simulink model "sus"  (Simulink 6.5)
settings: Solver=ode45  StartTime=0.0  StopTime=16  RelTol=1e-3
libraries: cdsFilt x266, cdsBitwise x92, cdsEpicsOut x84, cdsEpicsBinIn x56, cdsEpicsIn x20, cdsFiltCtrl x18, cdsMatrix x11, cdsSwitch x7, cdsWD x7, cdsFunctionCall x5, cdsRio1 x4, dac x3
(part 1 of 20)
settings Model: Creator=jay  LastModifiedBy=controls  ExtModeAutoUpdateStatusClock=off
settings DebuggingCC: MultiTaskDSMMsg=warning  MultiTaskCondExecSysMsg=none  StrictBusMsg=None
settings RTWCC: IncludeERTFirstTime=on

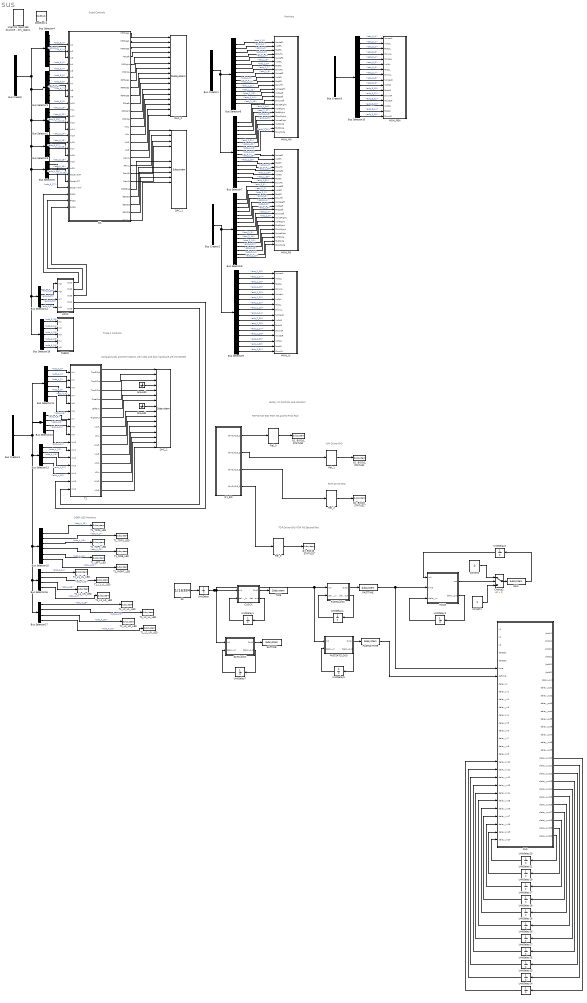
== system sus ==
  note: Quad Controls
  note: Monitors
  note: Binary IO Controls and Monitors
  note: UIM Driver BIO
  note: TOP Driver BIO FOR R0
      | Second Part
  note: PUM Driver BIO
  note: TOP Driver BIO FOR M0 and R0
      | First Part
  note: Triple 1 Controls
  note: Using grounds and terminators until ADC and DAC hardware are connected
  note: OSEM LED Monitors
  Bus Creator : BusCreator  Tag=adc_0  Description=|  Inputs='adc_0_0','adc_0_1','adc_0_2','adc_0_3','adc_0_4','adc_0_5','adc_0_6','adc_0_7','adc_0_8','adc_0_9','adc_0_10','adc_0_11','adc_0_12','adc_0_13','adc_0_14','adc_0_15','adc_0_16','adc_0_17','adc_0_18','adc_0_19','adc_0_20','adc_0_21','adc_0_22','adc_0_23','adc_0_24','adc_0_25','adc_0_26','adc_0_27','adc_0_28','adc_0_29','adc_0_30','adc_0_31'
      | PCI66-16AI64SSA
      | 40Vp-p, 16-bit, 610uV/count
      settings: AttributesFormatString=%<Description>\n%<Tag>
  Bus Creator1 : BusCreator  Tag=adc_1  Description=|  Inputs='adc_1_0','adc_1_1','adc_1_2','adc_1_3','adc_1_4','adc_1_5','adc_1_6','adc_1_7','adc_1_8','adc_1_9','adc_1_10','adc_1_11','adc_1_12','adc_1_13','adc_1_14','adc_1_15','adc_1_16','adc_1_17','adc_1_18','adc_1_19','adc_1_20','adc_1_21','adc_1_22','adc_1_23','adc_1_24','adc_1_25','adc_1_26','adc_1_27','adc_1_28','adc_1_29','adc_1_30','adc_1_31'
      | PCI66-16AI64SSA
      | 40Vp-p, 16-bit, 610uV/count
      settings: AttributesFormatString=%<Description>\n%<Tag>
  Bus Creator2 : BusCreator  Tag=adc_2  Description=|  Inputs='adc_2_0','adc_2_1','adc_2_2','adc_2_3','adc_2_4','adc_2_5','adc_2_6','adc_2_7','adc_2_8','adc_2_9','adc_2_10','adc_2_11','adc_2_12','adc_2_13','adc_2_14','adc_2_15','adc_2_16','adc_2_17','adc_2_18','adc_2_19','adc_2_20','adc_2_21','adc_2_22','adc_2_23','adc_2_24','adc_2_25','adc_2_26','adc_2_27','adc_2_28','adc_2_29','adc_2_30','adc_2_31'
      | PCI66-16AI64SSA
      | 40Vp-p, 16-bit, 610uV/count
      settings: AttributesFormatString=%<Description>\n%<Tag>
  Bus Creator3 : BusCreator  Tag=adc_3  Description=|  Inputs='adc_3_0','adc_3_1','adc_3_2','adc_3_3','adc_3_4','adc_3_5','adc_3_6','adc_3_7','adc_3_8','adc_3_9','adc_3_10','adc_3_11','adc_3_12','adc_3_13','adc_3_14','adc_3_15','adc_3_16','adc_3_17','adc_3_18','adc_3_19','adc_3_20','adc_3_21','adc_3_22','adc_3_23','adc_3_24','adc_3_25','adc_3_26','adc_3_27','adc_3_28','adc_3_29','adc_3_30','adc_3_31'
      | PCI66-16AI64SSA
      | 40Vp-p, 16-bit, 610uV/count
      settings: AttributesFormatString=%<Description>\n%<Tag>
  Bus Creator4 : BusCreator  Tag=adc_4  Description=|  Inputs='adc_4_0','adc_4_1','adc_4_2','adc_4_3','adc_4_4','adc_4_5','adc_4_6','adc_4_7','adc_4_8','adc_4_9','adc_4_10','adc_4_11','adc_4_12','adc_4_13','adc_4_14','adc_4_15','adc_4_16','adc_4_17','adc_4_18','adc_4_19','adc_4_20','adc_4_21','adc_4_22','adc_4_23','adc_4_24','adc_4_25','adc_4_26','adc_4_27','adc_4_28','adc_4_29','adc_4_30','adc_4_31'
      | PCI66-16AI64SSA
      | 40Vp-p, 16-bit, 610uV/count
      settings: AttributesFormatString=%<Description>\n%<Tag>
  Bus Selector1 : BusSelector  OutputSignals=adc_0_6,adc_0_7,adc_0_8,adc_0_9,adc_0_10,adc_0_11
  Bus Selector10 : BusSelector  OutputSignals=adc_3_0,adc_3_1,adc_3_2,adc_3_3,adc_3_4,adc_3_5,adc_3_6,adc_3_7,adc_3_8,adc_3_9,adc_3_10,adc_3_11,adc_3_12,adc_3_13,adc_3_14,adc_3_15
  Bus Selector11 : BusSelector  OutputSignals=adc_4_0,adc_4_1,adc_4_2,adc_4_4,adc_4_5,adc_4_6
  Bus Selector12 : BusSelector  OutputSignals=adc_4_8,adc_4_9,adc_4_10,adc_4_11
  Bus Selector13 : BusSelector  OutputSignals=adc_4_12,adc_4_13,adc_4_14,adc_4_15
  Bus Selector14 : BusSelector  OutputSignals=adc_0_18,adc_0_19,adc_0_20,adc_0_21
  Bus Selector15 : BusSelector  OutputSignals=adc_4_16,adc_4_17,adc_4_18,adc_4_20,adc_4_21,adc_4_22
  Bus Selector16 : BusSelector  OutputSignals=adc_4_24,adc_4_25,adc_4_26,adc_4_27
  Bus Selector17 : BusSelector  OutputSignals=adc_4_28,adc_4_29,adc_4_30,adc_4_31
  Bus Selector18 : BusSelector  OutputSignals=adc_0_20,adc_0_21,adc_0_22,adc_0_23,adc_0_24
  Bus Selector2 : BusSelector  OutputSignals=adc_0_12,adc_0_13,adc_0_14,adc_0_15
  Bus Selector3 : BusSelector  OutputSignals=adc_0_16,adc_0_17,adc_0_18,adc_0_19
  Bus Selector4 : BusSelector  OutputSignals=adc_0_0,adc_0_1,adc_0_2,adc_0_3,adc_0_4,adc_0_5
  Bus Selector5 : BusSelector  OutputSignals=adc_0_25,adc_0_26,adc_0_27
  Bus Selector6 : BusSelector  OutputSignals=adc_1_0,adc_1_1,adc_1_2,adc_1_3,adc_1_4,adc_1_5,adc_1_6,adc_1_7,adc_1_8,adc_1_9,adc_1_10,adc_1_11,adc_1_12,adc_1_13,adc_1_14,adc_1_15
  Bus Selector7 : BusSelector  OutputSignals=adc_1_16,adc_1_17,adc_1_18,adc_1_19,adc_1_20,adc_1_21,adc_1_22,adc_1_23,adc_1_24,adc_1_25,adc_1_26,adc_1_27,adc_1_28,adc_1_29,adc_1_30,adc_1_31
  Bus Selector8 : BusSelector  OutputSignals=adc_2_0,adc_2_1,adc_2_2,adc_2_3,adc_2_4,adc_2_5,adc_2_6,adc_2_7,adc_2_8,adc_2_9,adc_2_10,adc_2_11,adc_2_12,adc_2_13,adc_2_14,adc_2_15
  Bus Selector9 : BusSelector  OutputSignals=adc_2_16,adc_2_17,adc_2_18,adc_2_19,adc_2_20,adc_2_21,adc_2_22,adc_2_23,adc_2_24,adc_2_25,adc_2_26,adc_2_27,adc_2_28,adc_2_29,adc_2_30,adc_2_31
  CLOCK : Subsystem
  CONST1 : Constant
  CONST2 : Constant  Value=0
  Choice2 : Switch  Criteria=u2 > Threshold
  DAC_0 : dac/Subsystem  Tag=dac_0  Description=|  SystemSampleTime=-1
      | PCI66-16AO16
      | 20Vp-p, 16-bit, 305uV/count
      settings: AttributesFormatString=%<Description>
  DAC_1 : dac/Subsystem  Description=|  SystemSampleTime=-1
      | PCI66-16AO16
      | 20Vp-p, 16-bit, 305uV/count
      settings: AttributesFormatString=%<Description>
  DAC_2 : dac/Subsystem  Description=|  SystemSampleTime=-1
      | PCI66-16AO16
      | 20Vp-p, 16-bit, 305uV/count
      settings: AttributesFormatString=%<Description>
  DocBlock1 : simulink/Model-Wide Utilities/DocBlock  Tag=SW Install  SystemSampleTime=-1  DocumentType=Text
      settings: AttributesFormatString=%<Tag>
  FASTCLOCK : Subsystem
  FASTSATCLOCK : Subsystem
  FASTSATTIME : cdsFilt/Subsystem  Tag=cdsFilt  Description=|  SystemSampleTime=-1
      | Purpose:                                                                                                                                                                                                                                  
      | Standard CDS IIR filter module.                                                                                                                                                                                                           
      |                                                                                                                                                                                                                                           
      | Operation:                                                                                                                                                                                                                                
      | Consists of 10 second order section IIR filters, plus a ramped gain stage. In FE code, also provides pre-defined test points and excitation channel inputs. The filter coefficients are defined in the LIGO system using the 'foton' tool.
      |                                                                                                                                                                                                                                           
      | Usage:                                                                                                                                                                                                                                    
      | Name the part with the desired filter module name.
      settings: AttributesFormatString=%<Tag>
  FASTTIME : cdsFilt/Subsystem  Tag=cdsFilt  Description=|  SystemSampleTime=-1
      | Purpose:                                                                                                                                                                                                                                  
      | Standard CDS IIR filter module.                                                                                                                                                                                                           
      |                                                                                                                                                                                                                                           
      | Operation:                                                                                                                                                                                                                                
      | Consists of 10 second order section IIR filters, plus a ramped gain stage. In FE code, also provides pre-defined test points and excitation channel inputs. The filter coefficients are defined in the LIGO system using the 'foton' tool.
      |                                                                                                                                                                                                                                           
      | Usage:                                                                                                                                                                                                                                    
      | Name the part with the desired filter module name.
      settings: AttributesFormatString=%<Tag>
  Ground1 : Ground
  Ground2 : Ground
  HOLD : Subsystem
  LOCK : Subsystem
  MON_M0 : Subsystem
  MON_PEN : Subsystem
  MON_R0 : Subsystem
  MON_UI : Subsystem
  Q1 : Subsystem  Description=Quad Suspension
      settings: AttributesFormatString=%<Description>
  Q1_BIO16_STATUS0 : cdsEpicsOut/Subsystem  Tag=cdsEpicsOutput  Description=|  SystemSampleTime=-1
      | Purpose:                                          
      | Output a FE signal to an EPICS channel.           
      |                                                   
      | Operation:                                        
      | Takes input value and passes it to EPICS record.  
      |                                                   
      | Usage:                                            
      | Name the part with the desired EPICS rrecord name.
      settings: AttributesFormatString=%<Tag>
  Q1_BIO16_STATUS1 : cdsEpicsOut/Subsystem  Tag=cdsEpicsOutput  Description=|  SystemSampleTime=-1
      | Purpose:                                          
      | Output a FE signal to an EPICS channel.           
      |                                                   
      | Operation:                                        
      | Takes input value and passes it to EPICS record.  
      |                                                   
      | Usage:                                            
      | Name the part with the desired EPICS rrecord name.
      settings: AttributesFormatString=%<Tag>
  Q1_BIO16_STATUS2 : cdsEpicsOut/Subsystem  Tag=cdsEpicsOutput  Description=|  SystemSampleTime=-1
      | Purpose:                                          
      | Output a FE signal to an EPICS channel.           
      |                                                   
      | Operation:                                        
      | Takes input value and passes it to EPICS record.  
      |                                                   
      | Usage:                                            
      | Name the part with the desired EPICS rrecord name.
      settings: AttributesFormatString=%<Tag>
  Q1_BIO16_STATUS3 : cdsEpicsOut/Subsystem  Tag=cdsEpicsOutput  Description=|  SystemSampleTime=-1
      | Purpose:                                          
      | Output a FE signal to an EPICS channel.           
      |                                                   
      | Operation:                                        
      | Takes input value and passes it to EPICS record.  
      |                                                   
      | Usage:                                            
      | Name the part with the desired EPICS rrecord name.
      settings: AttributesFormatString=%<Tag>
  Q1_BO : Subsystem
  RLS : Subsystem
  Rel_{0..3} (4 alike) : cdsRio1/Subsystem  Tag=cdsRio1  Description=|  SystemSampleTime=-1
      | PCI IIRO 16 channel relay output
      | and isolated input module
      settings: AttributesFormatString=%<Tag>\n%<Description>
  SATCLOCK : Subsystem
  SATTIME : cdsFilt/Subsystem  Tag=cdsFilt  Description=|  SystemSampleTime=-1
      | Purpose:                                                                                                                                                                                                                                  
      | Standard CDS IIR filter module.                                                                                                                                                                                                           
      |                                                                                                                                                                                                                                           
      | Operation:                                                                                                                                                                                                                                
      | Consists of 10 second order section IIR filters, plus a ramped gain stage. In FE code, also provides pre-defined test points and excitation channel inputs. The filter coefficients are defined in the LIGO system using the 'foton' tool.
      |                                                                                                                                                                                                                                           
      | Usage:                                                                                                                                                                                                                                    
      | Name the part with the desired filter module name.
      settings: AttributesFormatString=%<Tag>
  SAW : cdsFilt/Subsystem  Tag=cdsFilt  Description=|  SystemSampleTime=-1
      | Purpose:                                                                                                                                                                                                                                  
      | Standard CDS IIR filter module.                                                                                                                                                                                                           
      |                                                                                                                                                                                                                                           
      | Operation:                                                                                                                                                                                                                                
      | Consists of 10 second order section IIR filters, plus a ramped gain stage. In FE code, also provides pre-defined test points and excitation channel inputs. The filter coefficients are defined in the LIGO system using the 'foton' tool.
      |                                                                                                                                                                                                                                           
      | Usage:                                                                                                                                                                                                                                    
      | Name the part with the desired filter module name.
      settings: AttributesFormatString=%<Tag>
  SR : Constant  Value=1/16384
  T1 : Subsystem  Description=Triple Suspension
      settings: AttributesFormatString=%<Description>
  T1_L1_LL_LED : cdsEpicsOut/Subsystem  Tag=cdsEpicsOutput  Description=|  SystemSampleTime=-1
      | Purpose:                                          
      | Output a FE signal to an EPICS channel.           
      |                                                   
      | Operation:                                        
      | Takes input value and passes it to EPICS record.  
      |                                                   
      | Usage:                                            
      | Name the part with the desired EPICS rrecord name.
      settings: AttributesFormatString=%<Tag>
  T1_L1_LR_LED : cdsEpicsOut/Subsystem  Tag=cdsEpicsOutput  Description=|  SystemSampleTime=-1
      | Purpose:                                          
      | Output a FE signal to an EPICS channel.           
      |                                                   
      | Operation:                                        
      | Takes input value and passes it to EPICS record.  
      |                                                   
      | Usage:                                            
      | Name the part with the desired EPICS rrecord name.
      settings: AttributesFormatString=%<Tag>
  T1_L1_UL_LED : cdsEpicsOut/Subsystem  Tag=cdsEpicsOutput  Description=|  SystemSampleTime=-1
      | Purpose:                                          
      | Output a FE signal to an EPICS channel.           
      |                                                   
      | Operation:                                        
      | Takes input value and passes it to EPICS record.  
      |                                                   
      | Usage:                                            
      | Name the part with the desired EPICS rrecord name.
      settings: AttributesFormatString=%<Tag>
  T1_L1_UR_LED : cdsEpicsOut/Subsystem  Tag=cdsEpicsOutput  Description=|  SystemSampleTime=-1
      | Purpose:                                          
      | Output a FE signal to an EPICS channel.           
      |                                                   
      | Operation:                                        
      | Takes input value and passes it to EPICS record.  
      |                                                   
      | Usage:                                            
      | Name the part with the desired EPICS rrecord name.
      settings: AttributesFormatString=%<Tag>
  T1_L2_LL_LED : cdsEpicsOut/Subsystem  Tag=cdsEpicsOutput  Description=|  SystemSampleTime=-1
      | Purpose:                                          
      | Output a FE signal to an EPICS channel.           
      |                                                   
      | Operation:                                        
      | Takes input value and passes it to EPICS record.  
      |                                                   
      | Usage:                                            
      | Name the part with the desired EPICS rrecord name.
      settings: AttributesFormatString=%<Tag>
  T1_L2_LR_LED : cdsEpicsOut/Subsystem  Tag=cdsEpicsOutput  Description=|  SystemSampleTime=-1
      | Purpose:                                          
      | Output a FE signal to an EPICS channel.           
      |                                                   
      | Operation:                                        
      | Takes input value and passes it to EPICS record.  
      |                                                   
      | Usage:                                            
      | Name the part with the desired EPICS rrecord name.
      settings: AttributesFormatString=%<Tag>
  T1_L2_UL_LED : cdsEpicsOut/Subsystem  Tag=cdsEpicsOutput  Description=|  SystemSampleTime=-1
      | Purpose:                                          
      | Output a FE signal to an EPICS channel.           
      |                                                   
      | Operation:                                        
      | Takes input value and passes it to EPICS record.  
      |                                                   
      | Usage:                                            
      | Name the part with the desired EPICS rrecord name.
      settings: AttributesFormatString=%<Tag>
  T1_L2_UR_LED : cdsEpicsOut/Subsystem  Tag=cdsEpicsOutput  Description=|  SystemSampleTime=-1
      | Purpose:                                          
      | Output a FE signal to an EPICS channel.           
      |                                                   
      | Operation:                                        
      | Takes input value and passes it to EPICS record.  
      |                                                   
      | Usage:                                            
      | Name the part with the desired EPICS rrecord name.
      settings: AttributesFormatString=%<Tag>
  T1_LEFT_LED : cdsEpicsOut/Subsystem  Tag=cdsEpicsOutput  Description=|  SystemSampleTime=-1
      | Purpose:                                          
      | Output a FE signal to an EPICS channel.           
      |                                                   
      | Operation:                                        
      | Takes input value and passes it to EPICS record.  
      |                                                   
      | Usage:                                            
      | Name the part with the desired EPICS rrecord name.
      settings: AttributesFormatString=%<Tag>
  T1_RIGHT_LED : cdsEpicsOut/Subsystem  Tag=cdsEpicsOutput  Description=|  SystemSampleTime=-1
      | Purpose:                                          
      | Output a FE signal to an EPICS channel.           
      |                                                   
      | Operation:                                        
      | Takes input value and passes it to EPICS record.  
      |                                                   
      | Usage:                                            
      | Name the part with the desired EPICS rrecord name.
      settings: AttributesFormatString=%<Tag>
  T1_SIDE_LED : cdsEpicsOut/Subsystem  Tag=cdsEpicsOutput  Description=|  SystemSampleTime=-1
      | Purpose:                                          
      | Output a FE signal to an EPICS channel.           
      |                                                   
      | Operation:                                        
      | Takes input value and passes it to EPICS record.  
      |                                                   
      | Usage:                                            
      | Name the part with the desired EPICS rrecord name.
      settings: AttributesFormatString=%<Tag>
  T1_TOP1_LED : cdsEpicsOut/Subsystem  Tag=cdsEpicsOutput  Description=|  SystemSampleTime=-1
      | Purpose:                                          
      | Output a FE signal to an EPICS channel.           
      |                                                   
      | Operation:                                        
      | Takes input value and passes it to EPICS record.  
      |                                                   
      | Usage:                                            
      | Name the part with the desired EPICS rrecord name.
      settings: AttributesFormatString=%<Tag>
  T1_TOP2_LED : cdsEpicsOut/Subsystem  Tag=cdsEpicsOutput  Description=|  SystemSampleTime=-1
      | Purpose:                                          
      | Output a FE signal to an EPICS channel.           
      |                                                   
      | Operation:                                        
      | Takes input value and passes it to EPICS record.  
      |                                                   
      | Usage:                                            
      | Name the part with the desired EPICS rrecord name.
      settings: AttributesFormatString=%<Tag>
  T1_TOP3_LED : cdsEpicsOut/Subsystem  Tag=cdsEpicsOutput  Description=|  SystemSampleTime=-1
      | Purpose:                                          
      | Output a FE signal to an EPICS channel.           
      |                                                   
      | Operation:                                        
      | Takes input value and passes it to EPICS record.  
      |                                                   
      | Usage:                                            
      | Name the part with the desired EPICS rrecord name.
      settings: AttributesFormatString=%<Tag>
  THERM : Subsystem
  TIME : cdsFilt/Subsystem  Tag=cdsFilt  Description=|  SystemSampleTime=-1
      | Purpose:                                                                                                                                                                                                                                  
      | Standard CDS IIR filter module.                                                                                                                                                                                                           
      |                                                                                                                                                                                                                                           
      | Operation:                                                                                                                                                                                                                                
      | Consists of 10 second order section IIR filters, plus a ramped gain stage. In FE code, also provides pre-defined test points and excitation channel inputs. The filter coefficients are defined in the LIGO system using the 'foton' tool.
      |                                                                                                                                                                                                                                           
      | Usage:                                                                                                                                                                                                                                    
      | Name the part with the desired filter module name.
      settings: AttributesFormatString=%<Tag>
  UnitDelay : UnitDelay
  UnitDelay{1..5,7,16..21,23..27} (17 alike) : UnitDelay  Orientation=left
  site=M1 rate=16K dcuid=9 gds_node_id=1 no_oversampling=1 no_dac_interpolation=1 shmem_daq=1 : cdsParameters/Subsystem  Tag=cdsParameters  SystemSampleTime=-1
      settings: AttributesFormatString=%<Tag>
  wires:
  Bus Selector4/1 -> Q1/1(In1)  "<adc_0_0>"
  Bus Selector4/2 -> Q1/2(In2)  "<adc_0_1>"
  Bus Selector4/3 -> Q1/3(In3)  "<adc_0_2>"
  Bus Selector4/4 -> Q1/4(In4)  "<adc_0_3>"
  Bus Selector4/5 -> Q1/5(In5)  "<adc_0_4>"
  Bus Selector4/6 -> Q1/6(In6)  "<adc_0_5>"
  Bus Selector1/1 -> Q1/7(In7)  "<adc_0_6>"
  Bus Selector1/2 -> Q1/8(In8)  "<adc_0_7>"
  Bus Selector1/3 -> Q1/9(In9)  "<adc_0_8>"
  Bus Selector1/6 -> Q1/12(In12)  "<adc_0_11>"
  Bus Selector1/5 -> Q1/11(In11)  "<adc_0_10>"
  Bus Selector1/4 -> Q1/10(In10)  "<adc_0_9>"
  Bus Selector2/1 -> Q1/13(In13)  "<adc_0_12>"
  Bus Selector2/2 -> Q1/14(In14)  "<adc_0_13>"
  Bus Selector2/3 -> Q1/15(In15)  "<adc_0_14>"
  Bus Selector2/4 -> Q1/16(In16)  "<adc_0_15>"
  Bus Creator/1 -> Bus Selector1/1, Bus Selector5/1, Bus Selector14/1, Bus Selector18/1, Bus Selector3/1, Bus Selector2/1, Bus Selector4/1
  Bus Selector3/1 -> Q1/17(In17)  "<adc_0_16>"
  Bus Selector3/2 -> Q1/18(In18)  "<adc_0_17>"
  Bus Selector3/3 -> Q1/19(In19)  "<adc_0_18>"
  Bus Selector3/4 -> Q1/20(In20)  "<adc_0_19>"
  Bus Creator1/1 -> Bus Selector6/1, Bus Selector7/1
  Bus Creator2/1 -> Bus Selector8/1, Bus Selector9/1
  Bus Creator3/1 -> Bus Selector10/1
  Rel_3/1 -> Q1_BIO16_STATUS3/1
  Rel_0/1 -> Q1_BIO16_STATUS0/1
  Rel_1/1 -> Q1_BIO16_STATUS1/1
  Bus Selector6/1 -> MON_M0/1(NoiseF1)  "<adc_1_0>"
  Bus Selector6/2 -> MON_M0/2(VoltF1)  "<adc_1_1>"
  Bus Selector6/3 -> MON_M0/3(FastF1)  "<adc_1_2>"
  Bus Selector6/4 -> MON_M0/4(SlowF1)  "<adc_1_3>"
  Bus Selector6/5 -> MON_M0/5(NoiseF2)  "<adc_1_4>"
  Bus Selector6/6 -> MON_M0/6(VoltF2)  "<adc_1_5>"
  Bus Selector6/7 -> MON_M0/7(FastF2)  "<adc_1_6>"
  Bus Selector6/8 -> MON_M0/8(SlowF2)  "<adc_1_7>"
  Bus Selector6/9 -> MON_M0/9(NoiseF3)  "<adc_1_8>"
  Bus Selector6/10 -> MON_M0/10(VoltF3)  "<adc_1_9>"
  Bus Selector6/11 -> MON_M0/11(FastF3)  "<adc_1_10>"
  Bus Selector6/12 -> MON_M0/12(SlowF3)  "<adc_1_11>"
  Bus Selector6/13 -> MON_M0/13(NoiseLeft)  "<adc_1_12>"
  Bus Selector6/14 -> MON_M0/14(VoltLeft)  "<adc_1_13>"
  Bus Selector6/15 -> MON_M0/15(FastLeft)  "<adc_1_14>"
  Bus Selector6/16 -> MON_M0/16(SlowLeft)  "<adc_1_15>"
  Bus Selector7/1 -> MON_M0/17(NoiseRight)  "<adc_1_16>"
  Bus Selector7/2 -> MON_M0/18(VoltRight)  "<adc_1_17>"
  Bus Selector7/3 -> MON_M0/19(FastRight)  "<adc_1_18>"
  Bus Selector7/4 -> MON_M0/20(SlowRight)  "<adc_1_19>"
  Bus Selector7/5 -> MON_M0/21(NoiseSide)  "<adc_1_20>"
  Bus Selector7/6 -> MON_M0/22(VoltSide)  "<adc_1_21>"
  Bus Selector7/7 -> MON_M0/23(FastSide)  "<adc_1_22>"
  Bus Selector7/8 -> MON_M0/24(SlowSide)  "<adc_1_23>"
  Bus Selector7/9 -> MON_R0/1(NoiseF1)  "<adc_1_24>"
  Bus Selector7/10 -> MON_R0/2(VoltF1)  "<adc_1_25>"
  Bus Selector7/11 -> MON_R0/3(FastF1)  "<adc_1_26>"
  Bus Selector7/12 -> MON_R0/4(SlowF1)  "<adc_1_27>"
  Bus Selector7/13 -> MON_R0/5(NoiseF2)  "<adc_1_28>"
  Bus Selector7/14 -> MON_R0/6(VoltF2)  "<adc_1_29>"
  Bus Selector7/15 -> MON_R0/7(FastF2)  "<adc_1_30>"
  Bus Selector7/16 -> MON_R0/8(SlowF2)  "<adc_1_31>"
  Bus Selector8/1 -> MON_R0/9(NoiseF3)  "<adc_2_0>"
  Bus Selector8/2 -> MON_R0/10(VoltF3)  "<adc_2_1>"
  Bus Selector8/3 -> MON_R0/11(FastF3)  "<adc_2_2>"
  Bus Selector8/4 -> MON_R0/12(SlowF3)  "<adc_2_3>"
  Bus Selector8/5 -> MON_R0/13(NoiseLeft)  "<adc_2_4>"
  Bus Selector8/6 -> MON_R0/14(VoltLeft)  "<adc_2_5>"
  Bus Selector8/7 -> MON_R0/15(FastLeft)  "<adc_2_6>"
  Bus Selector8/8 -> MON_R0/16(SlowLeft)  "<adc_2_7>"
  Bus Selector8/9 -> MON_R0/17(NoiseRight)  "<adc_2_8>"
  Bus Selector8/10 -> MON_R0/18(VoltRight)  "<adc_2_9>"
  Bus Selector8/11 -> MON_R0/19(FastRight)  "<adc_2_10>"
  Bus Selector8/12 -> MON_R0/20(SlowRight)  "<adc_2_11>"
  Bus Selector8/13 -> MON_R0/21(NoiseSide)  "<adc_2_12>"
  Bus Selector8/14 -> MON_R0/22(VoltSide)  "<adc_2_13>"
  Bus Selector8/15 -> MON_R0/23(FastSide)  "<adc_2_14>"
  Bus Selector8/16 -> MON_R0/24(SlowSide)  "<adc_2_15>"
  Bus Selector9/1 -> MON_UI/1(NoiseUL)  "<adc_2_16>"
  Bus Selector9/2 -> MON_UI/2(VoltUL)  "<adc_2_17>"
  Bus Selector9/3 -> MON_UI/3(FastUL)  "<adc_2_18>"
  Bus Selector9/4 -> MON_UI/4(SlowUL)  "<adc_2_19>"
  Bus Selector9/5 -> MON_UI/5(NoiseLL)  "<adc_2_20>"
  Bus Selector9/6 -> MON_UI/6(VoltLL)  "<adc_2_21>"
  Bus Selector9/7 -> MON_UI/7(FastLL)  "<adc_2_22>"
  Bus Selector9/8 -> MON_UI/8(SlowLL)  "<adc_2_23>"
  Bus Selector9/9 -> MON_UI/9(NoiseUR)  "<adc_2_24>"
  Bus Selector9/10 -> MON_UI/10(VoltUR)  "<adc_2_25>"
  Bus Selector9/11 -> MON_UI/11(FastUR)  "<adc_2_26>"
  Bus Selector9/12 -> MON_UI/12(SlowUR)  "<adc_2_27>"
  Bus Selector9/13 -> MON_UI/13(NoiseLR)  "<adc_2_28>"
  Bus Selector9/14 -> MON_UI/14(VoltLR)  "<adc_2_29>"
  Bus Selector9/15 -> MON_UI/15(FastLR)  "<adc_2_30>"
  Bus Selector9/16 -> MON_UI/16(SlowLR)  "<adc_2_31>"
  Bus Selector10/1 -> MON_PEN/1(NoiseUL)  "<adc_3_0>"
  Bus Selector10/2 -> MON_PEN/2(VoltUL)  "<adc_3_1>"
  Bus Selector10/3 -> MON_PEN/3(FastUL)  "<adc_3_2>"
  Bus Selector10/4 -> MON_PEN/4(SlowUL)  "<adc_3_3>"
  Bus Selector10/5 -> MON_PEN/5(NoiseLL)  "<adc_3_4>"
  Bus Selector10/6 -> MON_PEN/6(VoltLL)  "<adc_3_5>"
  Bus Selector10/7 -> MON_PEN/7(FastLL)  "<adc_3_6>"
  Bus Selector10/8 -> MON_PEN/8(SlowLL)  "<adc_3_7>"
  Bus Selector10/9 -> MON_PEN/9(NoiseUR)  "<adc_3_8>"
  Bus Selector10/10 -> MON_PEN/10(VoltUR)  "<adc_3_9>"
  Bus Selector10/11 -> MON_PEN/11(FastUR)  "<adc_3_10>"
  Bus Selector10/12 -> MON_PEN/12(SlowUR)  "<adc_3_11>"
  Bus Selector10/13 -> MON_PEN/13(NoiseLR)  "<adc_3_12>"
  Bus Selector10/14 -> MON_PEN/14(VoltLR)  "<adc_3_13>"
  Bus Selector10/15 -> MON_PEN/15(FastLR)  "<adc_3_14>"
  Bus Selector10/16 -> MON_PEN/16(SlowLR)  "<adc_3_15>"
  Q1/1(M0Face1) -> DAC_0/1
  Q1/2(M0Face2) -> DAC_0/2
  Q1/3(M0Face3) -> DAC_0/3
  Q1/4(M0Left) -> DAC_0/4
  Q1/5(M0Right) -> DAC_0/5
  Q1/6(M0Side) -> DAC_0/6
  Q1/7(R0Face1) -> DAC_0/7
  Q1/8(R0Face2) -> DAC_0/8
  Q1/9(R0Face3) -> DAC_0/9
  Q1/10(R0Left) -> DAC_0/10
  Q1/11(R0Right) -> DAC_0/11
  Q1/12(R0Side) -> DAC_0/12
  Q1/13(UIUL) -> DAC_0/13
  Q1/14(UILL) -> DAC_0/14
  Q1/15(UIUR) -> DAC_0/15
  Q1/16(UILR) -> DAC_0/16
  Q1/17(PenUL) -> DAC_1/1
  Q1/18(PenLL) -> DAC_1/2
  Q1/19(PenUR) -> DAC_1/3
  Q1/20(PenLR) -> DAC_1/4
  Q1/21(ESDBias) -> DAC_1/7
  Q1/22(ESDQ1) -> DAC_1/8
  Q1/23(ESDQ2) -> DAC_1/9
  Q1/24(ESDQ3) -> DAC_1/10
  Q1/25(ESDQ4) -> DAC_1/11
  Rel_2/1 -> Q1_BIO16_STATUS2/1
  Q1_BO/1(BinOut16_1) -> Rel_0/1
  Q1_BO/2(BinOut16_2) -> Rel_1/1
  Q1_BO/3(BinOut16_3) -> Rel_2/1
  Q1_BO/4(BinOut16_4) -> Rel_3/1
  Bus Selector14/1 -> LOCK/1(In5)  "<adc_0_28>"
  Bus Selector14/2 -> LOCK/2(In6)  "<adc_0_29>"
  Bus Selector14/3 -> LOCK/3(In7)  "<adc_0_30>"
  Bus Selector14/4 -> LOCK/4(In8)  "<adc_0_31>"
  LOCK/4(Out4) -> T1/15(In15)
  LOCK/5(Out5) -> T1/16(In16)
  LOCK/1(Out1) -> Q1/24(POS1)
  LOCK/2(Out2) -> Q1/25(POS2)
  LOCK/3(Out3) -> Q1/26(POS3)
  Bus Creator4/1 -> Bus Selector11/1, Bus Selector12/1, Bus Selector13/1, Bus Selector15/1, Bus Selector16/1, Bus Selector17/1
  Bus Selector11/1 -> T1/1(In1)  "<adc_4_0>"
  Bus Selector11/2 -> T1/2(In2)  "<adc_4_1>"
  Bus Selector11/3 -> T1/3(In3)  "<adc_4_2>"
  Bus Selector11/4 -> T1/4(In4)  "<adc_4_4>"
  Bus Selector11/5 -> T1/5(In5)  "<adc_4_5>"
  Bus Selector11/6 -> T1/6(In6)  "<adc_4_6>"
  Bus Selector12/1 -> T1/7(In7)  "<adc_4_8>"
  Bus Selector12/2 -> T1/8(In8)  "<adc_4_9>"
  Bus Selector12/3 -> T1/9(In9)  "<adc_4_10>"
  Bus Selector12/4 -> T1/10(In10)  "<adc_4_11>"
  Bus Selector13/1 -> T1/11(In11)  "<adc_4_12>"
  Bus Selector13/2 -> T1/12(In12)  "<adc_4_13>"
  Bus Selector13/3 -> T1/13(In13)  "<adc_4_14>"
  Bus Selector13/4 -> T1/14(In14)  "<adc_4_15>"
  Ground2/1 -> DAC_2/4
  T1/1(Top3Out) -> DAC_2/1
  T1/2(Top1Out) -> DAC_2/2
  T1/3(Top2Out) -> DAC_2/3
  Ground1/1 -> DAC_2/8
  T1/4(SideOut) -> DAC_2/5
  T1/5(LeftOut) -> DAC_2/6
  T1/6(RightOut) -> DAC_2/7
  T1/7(L1UL) -> DAC_2/9
  T1/8(L1LL) -> DAC_2/10
  T1/9(L1UR) -> DAC_2/11
  T1/10(L1LR) -> DAC_2/12
  T1/11(L2UL) -> DAC_2/13
  T1/12(L2LL) -> DAC_2/14
  T1/13(L2UR) -> DAC_2/15
  T1/14(L2LR) -> DAC_2/16
  Bus Selector15/1 -> T1_TOP3_LED/1  "<adc_4_16>"
  Bus Selector15/2 -> T1_TOP1_LED/1  "<adc_4_17>"
  Bus Selector15/3 -> T1_TOP2_LED/1  "<adc_4_18>"
  Bus Selector15/4 -> T1_SIDE_LED/1  "<adc_4_20>"
  Bus Selector15/5 -> T1_LEFT_LED/1  "<adc_4_21>"
  Bus Selector15/6 -> T1_RIGHT_LED/1  "<adc_4_22>"
  Bus Selector16/1 -> T1_L1_UL_LED/1  "<adc_4_24>"
  Bus Selector16/2 -> T1_L1_LL_LED/1  "<adc_4_25>"
  Bus Selector16/3 -> T1_L1_UR_LED/1  "<adc_4_26>"
  Bus Selector16/4 -> T1_L1_LR_LED/1  "<adc_4_27>"
  Bus Selector17/1 -> T1_L2_UL_LED/1  "<adc_4_28>"
  Bus Selector17/2 -> T1_L2_LL_LED/1  "<adc_4_29>"
  Bus Selector17/3 -> T1_L2_UR_LED/1  "<adc_4_30>"
  Bus Selector17/4 -> T1_L2_LR_LED/1  "<adc_4_31>"
  Bus Selector18/1 -> THERM/1(In1)  "<adc_0_20>"
  Bus Selector18/2 -> THERM/2(In2)  "<adc_0_21>"
  Bus Selector18/3 -> THERM/3(In3)  "<adc_0_22>"
  Bus Selector18/4 -> THERM/4(In4)  "<adc_0_23>"
  Bus Selector18/5 -> THERM/5(In5)  "<adc_0_24>"
  Bus Selector5/1 -> Q1/21(OpLevSUM)  "<adc_0_25>"
  Bus Selector5/2 -> Q1/22(OpLevPIT)  "<adc_0_26>"
  Bus Selector5/3 -> Q1/23(OpLevYAW)  "<adc_0_27>"
  CLOCK/1(Out1) -> TIME/1
  SR/1 -> UnitDelay/1
  UnitDelay/1 -> CLOCK/1(In1), SATCLOCK/1(In1), FASTCLOCK/1(In1), FASTSATCLOCK/1(In1)
  CLOCK/2(delay_out) -> UnitDelay1/1
  UnitDelay1/1 -> CLOCK/2(delay_in)
  SATCLOCK/2(delay_out) -> UnitDelay7/1
  UnitDelay7/1 -> SATCLOCK/2(delay_in)
  SATCLOCK/1(Out1) -> SATTIME/1
  HOLD/2(delay_out) -> UnitDelay2/1
  UnitDelay2/1 -> HOLD/3(delay_in)
  FASTTIME/1 -> HOLD/2(time), RLS/6(time)
  UnitDelay4/1 -> FASTCLOCK/2(delay_in)
  FASTCLOCK/1(Out1) -> FASTTIME/1
  FASTCLOCK/2(delay_out) -> UnitDelay4/1
  Choice2/1 -> SAW/1
  HOLD/1(out) -> Choice2/2
  CONST2/1 -> Choice2/1
  CONST1/1 -> Choice2/3
  SAW/1 -> UnitDelay3/1
  UnitDelay3/1 -> HOLD/1(In1)
  FASTSATCLOCK/2(delay_out) -> UnitDelay5/1
  UnitDelay5/1 -> FASTSATCLOCK/2(delay_in)
  FASTSATCLOCK/1(Out1) -> FASTSATTIME/1
  FASTSATTIME/1 -> RLS/7(sattime)
  UnitDelay20/1 -> RLS/28(delay_in20)
  UnitDelay21/1 -> RLS/27(delay_in19)
  UnitDelay19/1 -> RLS/26(delay_in18)
  UnitDelay17/1 -> RLS/25(delay_in17)
  UnitDelay18/1 -> RLS/24(delay_in16)
  UnitDelay16/1 -> RLS/23(delay_in15)
  UnitDelay26/1 -> RLS/22(delay_in14)
  UnitDelay27/1 -> RLS/21(delay_in13)
  UnitDelay25/1 -> RLS/20(delay_in12)
  UnitDelay23/1 -> RLS/19(delay_in11)
  UnitDelay24/1 -> RLS/18(delay_in10)
  RLS/27(delay_out20) -> UnitDelay20/1
  RLS/26(delay_out19) -> UnitDelay21/1
  RLS/25(delay_out18) -> UnitDelay19/1
  RLS/24(delay_out17) -> UnitDelay17/1
  RLS/23(delay_out16) -> UnitDelay18/1
  RLS/22(delay_out15) -> UnitDelay16/1
  RLS/21(delay_out14) -> UnitDelay26/1
  RLS/20(delay_out13) -> UnitDelay27/1
  RLS/19(delay_out12) -> UnitDelay25/1
  RLS/18(delay_out11) -> UnitDelay23/1
  RLS/17(delay_out10) -> UnitDelay24/1

== system sus/CLOCK ==
  In1 : Inport
  delay_in : Inport  Port=2
  CONST1 : Constant  Value=-94.5
  CONST2 : Constant  Value=0
  Choice2 : Switch  Threshold=94.5-(1/16384)
  Sum8 : Sum  Inputs=+++
  Out1 : Outport
  delay_out : Outport  Port=2
  wires:
  In1/1 -> Sum8/2
  Sum8/1 -> Out1/1, delay_out/1
  delay_in/1 -> Sum8/1, Choice2/2
  CONST1/1 -> Choice2/1
  CONST2/1 -> Choice2/3
  Choice2/1 -> Sum8/3

== system sus/FASTCLOCK ==
  In1 : Inport
  delay_in : Inport  Port=2
  CONST1 : Constant  Value=-0.5
  CONST2 : Constant  Value=0
  Choice2 : Switch  Threshold=0.5-(1/16384)
  Sum8 : Sum  Inputs=+++
  Out1 : Outport
  delay_out : Outport  Port=2
  wires:
  In1/1 -> Sum8/2
  Sum8/1 -> Out1/1, delay_out/1
  delay_in/1 -> Sum8/1, Choice2/2
  CONST1/1 -> Choice2/1
  CONST2/1 -> Choice2/3
  Choice2/1 -> Sum8/3

== system sus/FASTSATCLOCK ==
  In1 : Inport
  delay_in : Inport  Port=2
  Saturation : Saturate  UpperLimit=0.5+(1/16384)  LowerLimit=0
  Sum8 : Sum
  Out1 : Outport
  delay_out : Outport  Port=2
  wires:
  In1/1 -> Sum8/2
  Sum8/1 -> delay_out/1, Saturation/1
  delay_in/1 -> Sum8/1
  Saturation/1 -> Out1/1

== system sus/HOLD ==
  In1 : Inport
  time : Inport  Port=2
  delay_in : Inport  Port=3
  CONST1 : Constant  Orientation=left  Value=0
  CONST2 : Constant  Value=0
  Choice1 : Switch  Orientation=left  Threshold=0.5-(1/16384)
  Choice2 : Switch  Threshold=0.5-(1/16384)
  Gain1 : Gain
  Gain2 : Gain  Orientation=left  Gain=-1
  Sum8 : Sum  Inputs=+++
  out : Outport
  delay_out : Outport  Port=2
  wires:
  CONST2/1 -> Choice2/3
  time/1 -> Choice2/2, Choice1/2
  In1/1 -> Choice2/1
  Choice2/1 -> Sum8/2
  Sum8/1 -> delay_out/1
  delay_in/1 -> Gain2/1, Sum8/3, Gain1/1
  CONST1/1 -> Choice1/3
  Gain2/1 -> Choice1/1
  Choice1/1 -> Sum8/1
  Gain1/1 -> out/1
